simulink model "nls_flm"  (Simulink 6.3)
settings: Solver=ode23tb  StartTime=0.0  StopTime=3.0  RelTol=1e-3
values from neighbouring files (symbols this model uses):
  kf1 = 0.001    [init_flm.m]
  kf2 = 0.00001    (= 1e-05)    [init_flm.m]
  Tf11 = 0.5    [init_flm.m]
  Tf12 = 0.005    [init_flm.m]
  Tf21 = 1    [init_flm.m]
  Tf22 = 0.01    [init_flm.m]
undefined symbols (not defined in the file or in its folder): Ak, Bk, Ck, Dk
libraries: simulink x2
settings Model: LastModifiedBy=Petko Petkov  StrictBusMsg=None
settings DataIOCC: SignalLoggingName=sigsOut
settings OptimizationCC: BooleanDataType=off  InlineInvariantSignals=on
settings DebuggingCC: SolverPrmCheckMsg=none
settings HardwareCC: TargetUnknown=on
settings GRTTargetCC: ModelReferenceCompliant=off  MatFileLogging=off

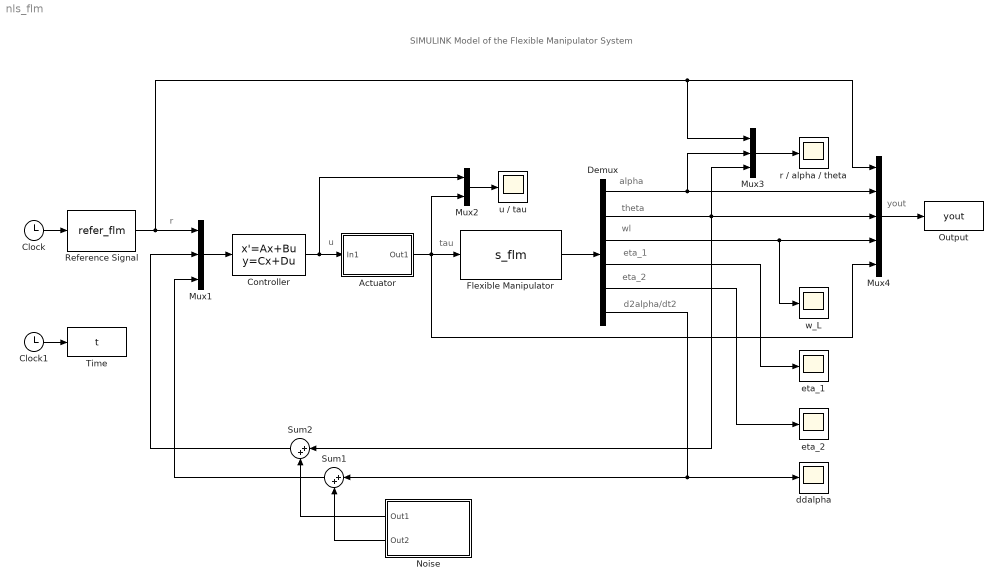
== system nls_flm ==
  note: SIMULINK Model of the Flexible Manipulator System
  note: alpha
  note: yout
  note: tau
  note: u
  note: r
  note: theta
  note: wl
  note: eta_1
  note: eta_2
  note: d2alpha/dt2
  Actuator : Subsystem
  Clock : Clock
  Clock1 : Clock
      settings: Decimation=10
  Controller : StateSpace  A=Ak  B=Bk  C=Ck  D=Dk
  Demux : Demux  Outputs=6
  Flexible Manipulator : S-Function  FunctionName=s_flm
  Mux1 : Mux  Inputs=3
  Mux2 : Mux  Inputs=2
  Mux3 : Mux  Inputs=3
  Mux4 : Mux  Inputs=5
  Noise : Subsystem  Orientation=left
  Output : ToWorkspace  VariableName=yout  SampleTime=-1  SaveFormat=Array
  Reference Signal : S-Function  FunctionName=refer_flm
  Sum1 : Sum  Orientation=left  Inputs=|++  SaturateOnIntegerOverflow=on  InputSameDT=on
  Sum2 : Sum  Orientation=left  Inputs=|++  SaturateOnIntegerOverflow=on  InputSameDT=on
  Time : ToWorkspace  VariableName=t  SampleTime=-1  SaveFormat=Array
  ddalpha : Scope
      settings: YMin=-0.225  YMax=0.15  SaveName=ScopeData4  MaxDataPoints=10000
  eta_1 : Scope
      settings: YMin=-0.225  YMax=0.15  SaveName=ScopeData2  MaxDataPoints=10000
  eta_2 : Scope
      settings: YMin=-0.225  YMax=0.15  SaveName=ScopeData3  MaxDataPoints=10000
  r / alpha / theta : Scope
      settings: YMin=-0.025  YMax=0.275  SaveName=ScopeData6  MaxDataPoints=10000
  u / tau : Scope
      settings: YMin=-3.5  YMax=6  MaxDataPoints=10000
  w_L : Scope
      settings: YMin=-3.5e-005  YMax=4e-005  MaxDataPoints=10000
  wires:
  Flexible Manipulator/1 -> Demux/1
  Clock/1 -> Reference Signal/1
  Clock1/1 -> Time/1
  Mux2/1 -> u / tau/1
  Mux3/1 -> r / alpha / theta/1
  Mux4/1 -> Output/1
  Demux/1 -> Mux4/2, Mux3/2
  Reference Signal/1 -> Mux4/1, Mux3/1, Mux1/1
  Actuator/1(Out1) -> Flexible Manipulator/1, Mux2/2, Mux4/5
  Noise/1(Out1) -> Sum2/2
  Noise/2(Out2) -> Sum1/2
  Mux1/1 -> Controller/1
  Controller/1 -> Actuator/1(In1), Mux2/1
  Sum2/1 -> Mux1/2
  Sum1/1 -> Mux1/3
  Demux/2 -> Mux3/3, Mux4/3, Sum2/1
  Demux/6 -> Sum1/1, ddalpha/1
  Demux/3 -> Mux4/4, w_L/1
  Demux/4 -> eta_1/1
  Demux/5 -> eta_2/1

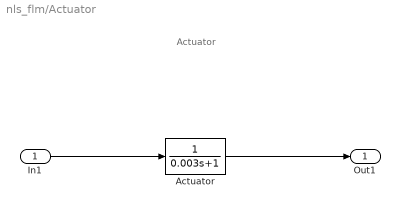
== system nls_flm/Actuator ==
  note: Actuator
  In1 : Inport
  Actuator : TransferFcn  Denominator="[0.003  1]"
  Out1 : Outport
  wires:
  In1/1 -> Actuator/1
  Actuator/1 -> Out1/1

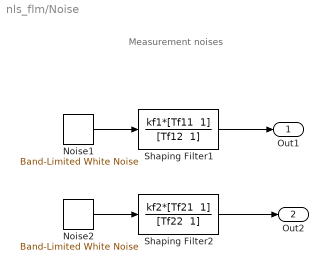
== system nls_flm/Noise ==
  note: Measurement noises
  Noise1 : simulink/Sources/Band-Limited White Noise  Cov=10^(-6)  Ts=0.2  seed=[23341]
  Noise2 : simulink/Sources/Band-Limited White Noise  Cov=10^(-6)  Ts=0.2  seed=[23341]
  Shaping Filter1 : TransferFcn  Numerator="kf1*[Tf11  1]"  Denominator="[Tf12  1]"
  Shaping Filter2 : TransferFcn  Numerator="kf2*[Tf21  1]"  Denominator="[Tf22  1]"
  Out1 : Outport
  Out2 : Outport  Port=2
  wires:
  Noise1/1 -> Shaping Filter1/1
  Shaping Filter1/1 -> Out1/1
  Noise2/1 -> Shaping Filter2/1
  Shaping Filter2/1 -> Out2/1
